simulink model "test_filter"  (R2020a)
settings: Solver=VariableStepAuto  StartTime=0.0  StopTime=10.0  RelTol=1e-3
values from neighbouring files (symbols this model uses):
  Af = [0 1; -w^2 -2*w]    [init_oscillator_2021_03_26.m]
  Afd = [exp(-Ts*w)*(1+Ts*w) exp(-Ts*w)*Ts; -exp(-Ts*w)*Ts*w^2 exp(-Ts*w)*(1-Ts*w)]    [init_oscillator_2021_03_26.m]
  Bf = [0 1]'    [init_oscillator_2021_03_26.m]
  Bfd = [(1-exp(-Ts*w)*(1+Ts*w))/w^2 exp(-Ts*w)*Ts]'    [init_oscillator_2021_03_26.m]
  Cf = [2*w^2 0]    [init_oscillator_2021_03_26.m]
  Ts = 1/20e3    (= 5e-05)    [init_oscillator_2021_03_26.m]
  w = 2*pi*f    (= 1570.79632679)    [init_oscillator_2021_03_26.m]
settings Model: Creator=dbagn  LastModifiedBy=dbagn

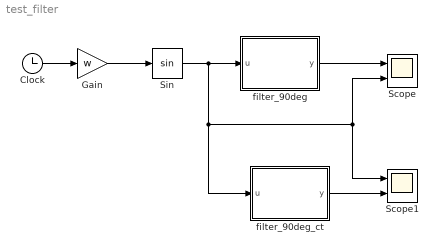
== system test_filter ==
  Clock : Clock
  Gain : Gain  Gain=w
  Scope : Scope  NumInputPorts=2
  Scope1 : Scope  NumInputPorts=2
  Sin : Trigonometry
  filter_90deg : Subsystem
  filter_90deg_ct : Subsystem
  wires:
  Clock/1 -> Gain/1
  Gain/1 -> Sin/1
  Sin/1 -> filter_90deg_ct/1(u), Scope/2, Scope1/1, filter_90deg/1(u)
  filter_90deg/1(y) -> Scope/1
  filter_90deg_ct/1(y) -> Scope1/2

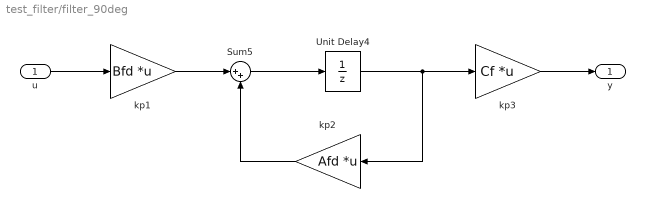
== system test_filter/filter_90deg ==
  u : Inport
  Sum5 : Sum  Inputs=|++
  Unit Delay4 : UnitDelay  SampleTime=Ts  HasFrameUpgradeWarning=on
  kp1 : Gain  Gain=Bfd  Multiplication=Matrix(K*u)  SaturateOnIntegerOverflow=on  OutDataTypeStr=Inherit: Same as input  ParamDataTypeStr=Inherit: Same as input
  kp2 : Gain  Gain=Afd  Multiplication=Matrix(K*u)  SaturateOnIntegerOverflow=on  OutDataTypeStr=Inherit: Same as input  ParamDataTypeStr=Inherit: Same as input
  kp3 : Gain  Gain=Cf  Multiplication=Matrix(K*u)  SaturateOnIntegerOverflow=on  OutDataTypeStr=Inherit: Same as input  ParamDataTypeStr=Inherit: Same as input
  y : Outport
  wires:
  Unit Delay4/1 -> kp2/1, kp3/1
  Sum5/1 -> Unit Delay4/1
  kp2/1 -> Sum5/2
  kp1/1 -> Sum5/1
  u/1 -> kp1/1
  kp3/1 -> y/1

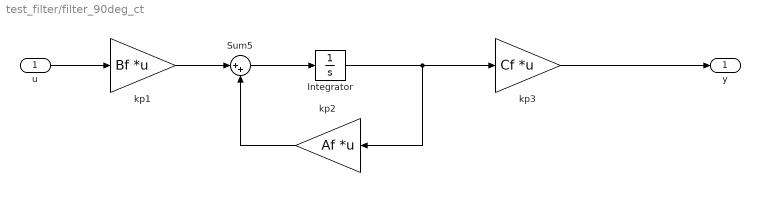
== system test_filter/filter_90deg_ct ==
  u : Inport
  Integrator : Integrator
  Sum5 : Sum  Inputs=|++
  kp1 : Gain  Gain=Bf  Multiplication=Matrix(K*u)  SaturateOnIntegerOverflow=on  OutDataTypeStr=Inherit: Same as input  ParamDataTypeStr=Inherit: Same as input
  kp2 : Gain  Gain=Af  Multiplication=Matrix(K*u)  SaturateOnIntegerOverflow=on  OutDataTypeStr=Inherit: Same as input  ParamDataTypeStr=Inherit: Same as input
  kp3 : Gain  Gain=Cf  Multiplication=Matrix(K*u)  SaturateOnIntegerOverflow=on  OutDataTypeStr=Inherit: Same as input  ParamDataTypeStr=Inherit: Same as input
  y : Outport
  wires:
  kp3/1 -> y/1
  u/1 -> kp1/1
  kp1/1 -> Sum5/1
  kp2/1 -> Sum5/2
  Sum5/1 -> Integrator/1
  Integrator/1 -> kp3/1, kp2/1
